simulink model "instabile"  (R2022b)
settings: Solver=VariableStepAuto  StartTime=0.0  StopTime=10.0  RelTol=1e-3
values from neighbouring files (symbols this model uses):
  K = linspace(0.01,0.2,7)    [untitled.m]    (also in untitled2.m)
  sys1 = tf(num,den)    [untitled.m]    (also in untitled2.m)
undefined symbols (not defined in the file or in its folder): i
settings Model: Creator=danie  LastModifiedBy=danie

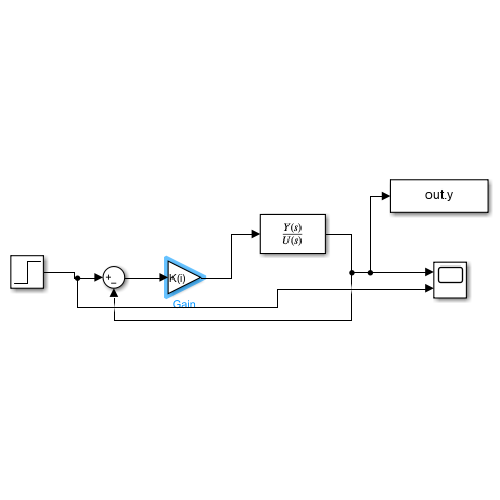
[thumbnail: Simulink's stored preview of the top-level diagram]
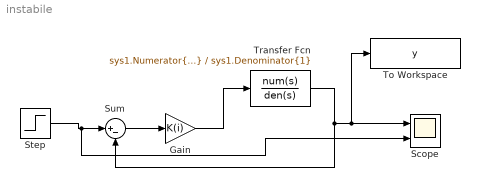
== system instabile ==
  Gain : Gain  Gain=K(i)
  Scope : Scope  NumInputPorts=2
  Step : Step  SampleTime=0
  Sum : Sum  Inputs=|+-
  To Workspace : ToWorkspace  VariableName=y  SaveFormat=Timeseries  SampleTime=-1
  Transfer Fcn : TransferFcn  Numerator=sys1.Numerator{1}  Denominator=sys1.Denominator{1}
  wires:
  Gain/1 -> Transfer Fcn/1
  Sum/1 -> Gain/1
  Transfer Fcn/1 -> Sum/2, To Workspace/1, Scope/1
  Step/1 -> Scope/2, Sum/1
